simulink model "rtwdemo_mrmtbb"  (Simulink 7.6)
settings: Solver=FixedStepDiscrete  SolverMode=MultiTasking  StartTime=0.0  StopTime=10.0  RelTol=1e-3  SampleTimeConstraint=Specified
undefined symbols (not defined in the file or in its folder): DiscIntNeverNeededParam
libraries: rtwdemowidgets x4
Description:
  | Multirate Modeling in Multitasking Mode (Bare Board, no OS)
settings Model: Creator=The MathWorks Inc.  ExtModeArmWhenConnect=off  ExtModeAutoUpdateStatusClock=off
settings MATStruct: SampleTime=1  Offset=0  Priority=[0.0]
settings DataIOCC: SaveOutput=off  SaveTime=off  SignalLoggingName=sigsOut
settings OptimizationCC: InlineParams=on  InlineInvariantSignals=on  StateBitsets=on  DataBitsets=on  UseTempVars=on  EfficientFloat2IntCast=on  EfficientMapNaN2IntZero=off
settings DebuggingCC: CheckExecutionContextPreStartOutputMsg=on  CheckExecutionContextRuntimeOutputMsg=on  SolverPrmCheckMsg=none  UnconnectedInputMsg=none  UnconnectedOutputMsg=none  UnconnectedLineMsg=none  StrictBusMsg=ErrorOnBusTreatedAsVector
settings HardwareCC: ProdIntDivRoundTo=Zero  ProdEndianess=LittleEndian  ProdHWDeviceType=Generic->32-bit Embedded Processor  TargetHWDeviceType=Generic->32-bit Embedded Processor
settings ModelReferenceCC: UpdateModelReferenceTargets=IfOutOfDate
settings RTWCC: TLCOptions=-p0 -aWarnNonSaturatedBlocks=0  GenerateReport=on  RTWVerbose=off  ProcessScript=grt_make_rtw_hook  LaunchReport=on
settings CodeAppCC: ForceParamTrailComments=on
settings GRTTargetCC: TargetFcnLib=ansi_tfl_tmw.mat

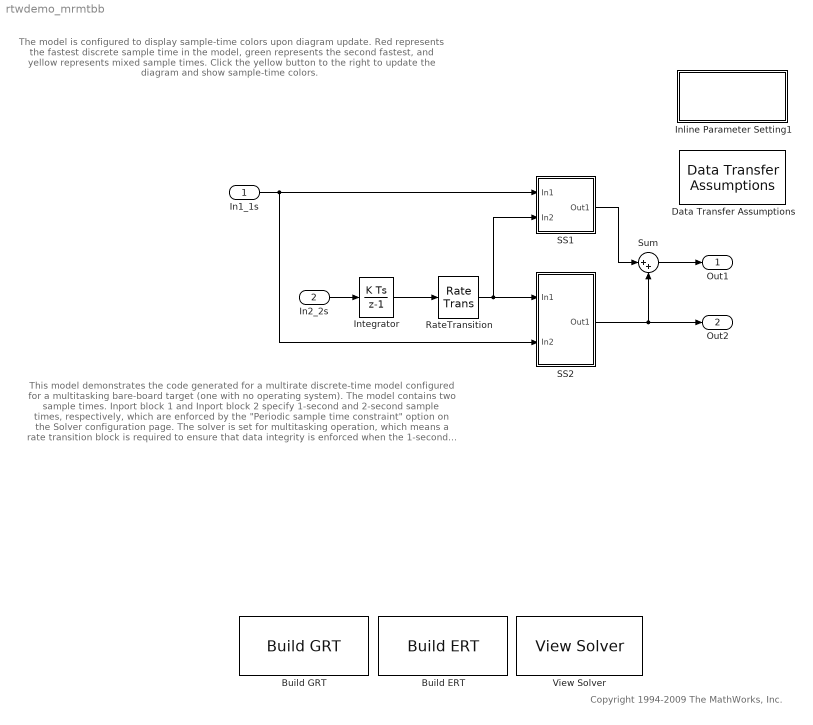
== system rtwdemo_mrmtbb ==
  note: This model demonstrates the code generated for a multirate discrete-time model
      | configured for a multitasking bare-board target (one with no operating system).  The
      | model contains two sample times.  Inport block 1 and Inport block 2 specify 1-second
      | and 2-second sample times, respectively, which are enforced by the "Periodic
      | sample time constraint" option on the Solver configuration page.  The solver is set for
      | multitasking operation, which means a rate transition block is required to ensure that
      | data integrity is enforced when the 1-second task preempts the 2-second task.
      | Proper rate transitions are always enforced by Simulink and Real-Time Workshop.
      | This model specifies an explicit rate transition block.  Alternatively, this block could
      | be automatically inserted by Simulink using the "Automatically handle data transfers
      | between tasks" option on the Solver configuration page.
  note: The model is configured to display sample-time colors upon
      | diagram update.  Red represents the fastest discrete sample
      | time in the model, green represents the second fastest, and
      | yellow represents mixed sample times.  Click the yellow button
      | to the right to update the diagram and show sample-time colors.
  note: Copyright 1994-2009 The MathWorks, Inc.
  In1_1s : Inport  OutDataTypeStr=double  PortDimensions=1  SampleTime=1
  In2_2s : Inport  Port=2  OutDataTypeStr=double  PortDimensions=1  SampleTime=2
  Build ERT : rtwdemowidgets/Build ERT  SystemSampleTime=-1  attrib_overrides={}
  Build GRT : rtwdemowidgets/Build GRT  SystemSampleTime=-1  attrib_overrides={}
  Data Transfer Assumptions : rtwdemowidgets/Data Transfer Assumptions  SystemSampleTime=-1
  Inline Parameter Setting1 : Subsystem
      settings: OpenFcn=m=get_param(bdroot,'name'); set_param(bdroot, 'SampleTimeColors','on'); eval([m,'([],[],[],''compile'');']); eval([m,'([],[],[],''term'');']);clear m;
      mask Display: disp(sprintf('Display Sample\nTime Colors\n(double-click)'))
  Integrator : DiscreteIntegrator  InitialConditionMode=State only (most efficient)  SampleTime=-1  SaturateOnIntegerOverflow=on  ICPrevOutput=DiscIntNeverNeededParam  ICPrevScaledInput=DiscIntNeverNeededParam
  RateTransition : RateTransition
  SS1 : Subsystem  TreatAsAtomicUnit=on
  SS2 : Subsystem  TreatAsAtomicUnit=on
  Sum : Sum  Inputs=|++  SaturateOnIntegerOverflow=on  InputSameDT=on  OutDataTypeStr=Inherit: Same as first input
  View Solver : rtwdemowidgets/View Solver  SystemSampleTime=-1
  Out1 : Outport
  Out2 : Outport  Port=2
  wires:
  In1_1s/1 -> SS1/1(In1), SS2/2(In2)
  In2_2s/1 -> Integrator/1
  SS2/1(Out1) -> Out2/1, Sum/2
  SS1/1(Out1) -> Sum/1
  Sum/1 -> Out1/1
  RateTransition/1 -> SS2/1(In1), SS1/2(In2)
  Integrator/1 -> RateTransition/1

== system rtwdemo_mrmtbb/Inline Parameter Setting1 ==

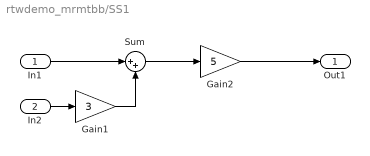
== system rtwdemo_mrmtbb/SS1 ==
  In1 : Inport
  In2 : Inport  Port=2
  Gain1 : Gain  Gain=3  SaturateOnIntegerOverflow=on  OutDataTypeStr=Inherit: Same as input  ParamDataTypeStr=Inherit: Same as input
  Gain2 : Gain  Gain=5  SaturateOnIntegerOverflow=on  OutDataTypeStr=Inherit: Same as input  ParamDataTypeStr=Inherit: Same as input
  Sum : Sum  Inputs=|++  SaturateOnIntegerOverflow=on  InputSameDT=on  OutDataTypeStr=Inherit: Same as first input
  Out1 : Outport
  wires:
  In1/1 -> Sum/1
  Sum/1 -> Gain2/1
  In2/1 -> Gain1/1
  Gain2/1 -> Out1/1
  Gain1/1 -> Sum/2

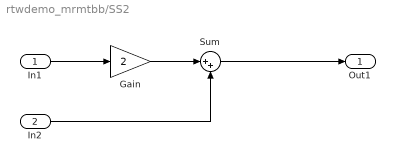
== system rtwdemo_mrmtbb/SS2 ==
  In1 : Inport
  In2 : Inport  Port=2
  Gain : Gain  Gain=2  SaturateOnIntegerOverflow=on  OutDataTypeStr=Inherit: Same as input  ParamDataTypeStr=Inherit: Same as input
  Sum : Sum  Inputs=|++  SaturateOnIntegerOverflow=on  InputSameDT=on  OutDataTypeStr=Inherit: Same as first input
  Out1 : Outport
  wires:
  In1/1 -> Gain/1
  Gain/1 -> Sum/1
  Sum/1 -> Out1/1
  In2/1 -> Sum/2
